simulink model "Leg_Torque_Controls"  (R2018b)
settings: Solver=VariableStepAuto  StartTime=0.0  StopTime=10.0  RelTol=1e-3
settings Model: Creator=Nathan Boyd  LastModifiedBy=Nathan Boyd

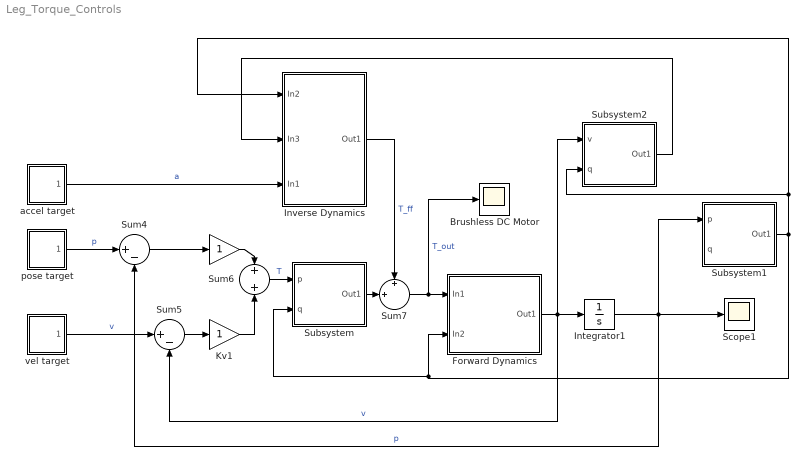
== system Leg_Torque_Controls ==
  " " : Gain
  " accel target" : Subsystem
  " vel target" : Subsystem
  Brushless DC Motor : Scope
  Forward Dynamics : Subsystem
  Integrator1 : Integrator
  Inverse Dynamics : Subsystem
  Kv1 : Gain
  Scope1 : Scope
  Subsystem : Subsystem
  Subsystem1 : Subsystem
  Subsystem2 : Subsystem
  Sum4 : Sum  Inputs=|+-
  Sum5 : Sum  Inputs=|+-
  Sum6 : Sum
  Sum7 : Sum  Inputs=+|+||
  pose target : Subsystem
  wires:
  Inverse Dynamics/1(Out1) -> Sum7/1  "T_ff"
  Integrator1/1 -> Sum4/2, Scope1/1, Subsystem1/1(p)  "p"
  pose target/1(Out1) -> Sum4/1  "p"
  Sum4/1 -> " "/1
  Sum7/1 -> Brushless DC Motor/1, Forward Dynamics/1(In1)  "T_out"
  Kv1/1 -> Sum6/2
  " accel target"/1(Out1) -> Inverse Dynamics/3(In1)  "a"
  Forward Dynamics/1(Out1) -> Subsystem2/1(v), Integrator1/1, Sum5/2  "v"
  " "/1 -> Sum6/1
  Sum5/1 -> Kv1/1
  " vel target"/1(Out1) -> Sum5/1  "v"
  Sum6/1 -> Subsystem/1(p)  "T"
  Subsystem/1(Out1) -> Sum7/2
  Subsystem1/1(Out1) -> Subsystem/2(q), Forward Dynamics/2(In2), Inverse Dynamics/1(In2), Subsystem2/2(q)
  Subsystem2/1(Out1) -> Inverse Dynamics/2(In3)

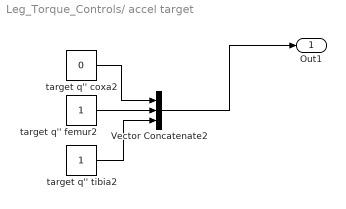
== system Leg_Torque_Controls/ accel target ==
  Vector Concatenate2 : Concatenate  NumInputs=3
  target q'' coxa2 : Constant  Value=0
  target q'' femur2 : Constant
  target q'' tibia2 : Constant
  Out1 : Outport
  wires:
  target q'' tibia2/1 -> Vector Concatenate2/3
  target q'' femur2/1 -> Vector Concatenate2/2
  target q'' coxa2/1 -> Vector Concatenate2/1
  Vector Concatenate2/1 -> Out1/1

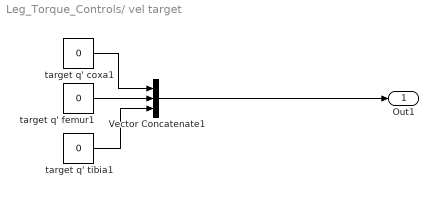
== system Leg_Torque_Controls/ vel target ==
  Vector Concatenate1 : Concatenate  NumInputs=3
  target q' coxa1 : Constant  Value=0
  target q' femur1 : Constant  Value=0
  target q' tibia1 : Constant  Value=0
  Out1 : Outport
  wires:
  target q' femur1/1 -> Vector Concatenate1/2
  target q' coxa1/1 -> Vector Concatenate1/1
  target q' tibia1/1 -> Vector Concatenate1/3
  Vector Concatenate1/1 -> Out1/1

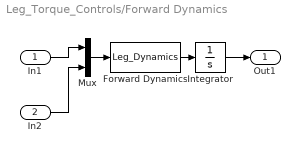
== system Leg_Torque_Controls/Forward Dynamics ==
  In1 : Inport
  In2 : Inport  Port=2
  Forward Dynamics : MATLABFcn  MATLABFcn=Leg_Dynamics
  Integrator : Integrator
  Mux : Mux  Inputs=2
  Out1 : Outport
  wires:
  Forward Dynamics/1 -> Integrator/1
  In1/1 -> Mux/1
  Integrator/1 -> Out1/1
  In2/1 -> Mux/2
  Mux/1 -> Forward Dynamics/1

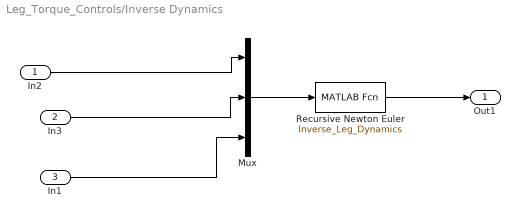
== system Leg_Torque_Controls/Inverse Dynamics ==
  In2 : Inport
  In3 : Inport  Port=2
  In1 : Inport  Port=3
  Mux : Mux  Inputs=3
  Recursive Newton Euler : MATLABFcn  MATLABFcn=Inverse_Leg_Dynamics
  Out1 : Outport
  wires:
  Mux/1 -> Recursive Newton Euler/1
  Recursive Newton Euler/1 -> Out1/1
  In1/1 -> Mux/3
  In2/1 -> Mux/1
  In3/1 -> Mux/2

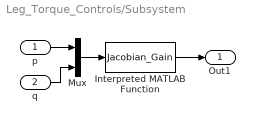
== system Leg_Torque_Controls/Subsystem ==
  p : Inport
  q : Inport  Port=2
  Interpreted MATLAB Function : MATLABFcn  MATLABFcn=Jacobian_Gain
  Mux : Mux  Inputs=2
  Out1 : Outport
  wires:
  p/1 -> Mux/1
  Interpreted MATLAB Function/1 -> Out1/1
  q/1 -> Mux/2
  Mux/1 -> Interpreted MATLAB Function/1

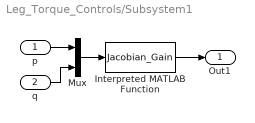
== system Leg_Torque_Controls/Subsystem1 ==
  p : Inport
  q : Inport  Port=2
  Interpreted MATLAB Function : MATLABFcn  MATLABFcn=Jacobian_Gain
  Mux : Mux  Inputs=2
  Out1 : Outport
  wires:
  p/1 -> Mux/1
  Interpreted MATLAB Function/1 -> Out1/1
  q/1 -> Mux/2
  Mux/1 -> Interpreted MATLAB Function/1

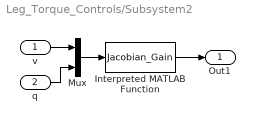
== system Leg_Torque_Controls/Subsystem2 ==
  v : Inport
  q : Inport  Port=2
  Interpreted MATLAB Function : MATLABFcn  MATLABFcn=Jacobian_Gain
  Mux : Mux  Inputs=2
  Out1 : Outport
  wires:
  v/1 -> Mux/1
  Interpreted MATLAB Function/1 -> Out1/1
  q/1 -> Mux/2
  Mux/1 -> Interpreted MATLAB Function/1

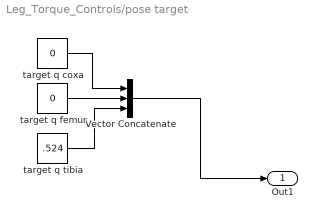
== system Leg_Torque_Controls/pose target ==
  Vector Concatenate : Concatenate  NumInputs=3
  target q coxa : Constant  Value=0
  target q femur : Constant  Value=0
  target q tibia : Constant  Value=.524
  Out1 : Outport
  wires:
  target q coxa/1 -> Vector Concatenate/1
  Vector Concatenate/1 -> Out1/1
  target q femur/1 -> Vector Concatenate/2
  target q tibia/1 -> Vector Concatenate/3
